simulink model "nlarx_ROM"  (R2025a)
settings: Solver=VariableStepAuto  StartTime=0.0  StopTime=5000  FixedStep=0.1  RelTol=1e-3
libraries: slident x1
settings Model: SimulationMode=accelerator  Creator=The MathWorks, Inc.  LastModifiedBy=skeshavm
settings OptimizationCC: ReuseModelBlockBuffer=off
settings DebuggingCC: UnconnectedInputMsg=warning  UnconnectedOutputMsg=warning  UnconnectedLineMsg=warning
settings ModelReferenceCC: EnableRefExpFcnMdlSchedulingChecks=on
settings RTWCC: GPUComputeCapability=3.5  DLArmComputeVersion=19.05

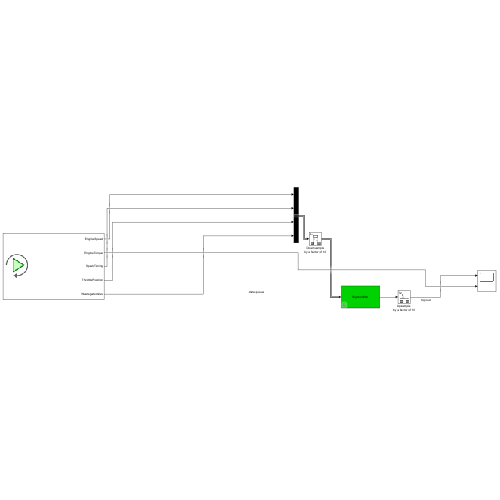
[thumbnail: Simulink's stored preview of the top-level diagram]
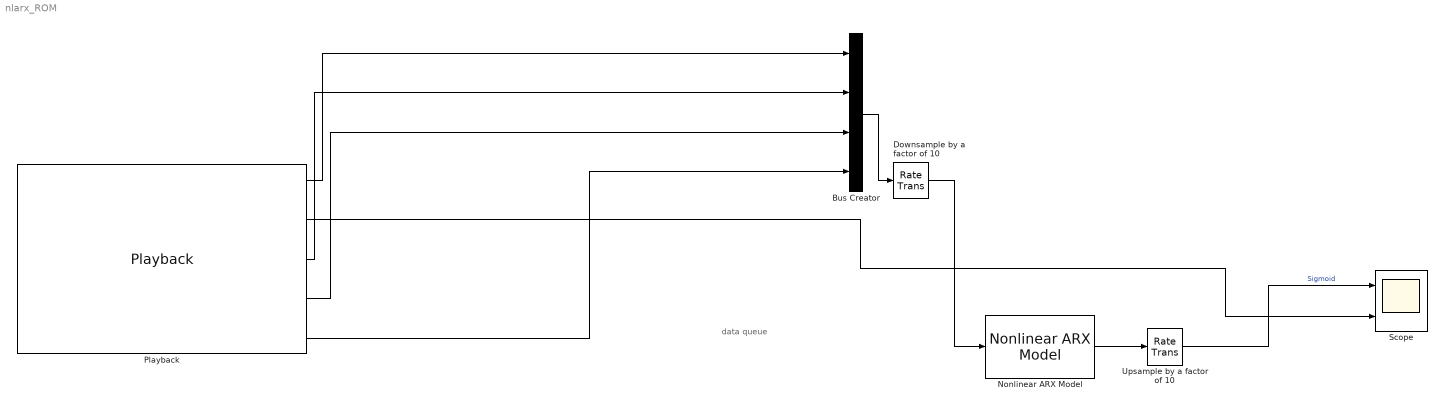
== system nlarx_ROM ==
  note: data queue
  Bus Creator : BusCreator  Inputs=4
  Downsample by a factor of 10 : RateTransition  Deterministic=off  OutPortSampleTime=1
  Nonlinear ARX Model : slident/Models/Nonlinear ARX Model  sys=SigmoidNet  ICspec=Input and output values  X0=0  U0=0  Y0=0
  Playback : Playback  NumPorts=5  PartName=bf1491cc-dadc-4842-a20c-aa9ee90bf378  TablePosition=Bottom
  Scope : Scope  NumInputPorts=2
      settings: ActiveDisplayYMinimum=-473.35707172439538  ActiveDisplayYMaximum=4260.21364551956
  Upsample by a factor of 10 : RateTransition  OutPortSampleTime=0.1
  wires:
  Downsample by a factor of 10/1 -> Nonlinear ARX Model/1
  Upsample by a factor of 10/1 -> Scope/1  "Sigmoid"
  Nonlinear ARX Model/1 -> Upsample by a factor of 10/1
  Playback/2 -> Scope/2
  Bus Creator/1 -> Downsample by a factor of 10/1
  Playback/1 -> Bus Creator/1
  Playback/3 -> Bus Creator/2
  Playback/4 -> Bus Creator/3
  Playback/5 -> Bus Creator/4
